simulink model "Project_000481137"  (R2022b)
settings: Solver=VariableStepAuto  StartTime=0.0  StopTime=10.0  RelTol=1e-3
values from neighbouring files (symbols this model uses):
  a1 = 0.3102    [Constants.m]
  A1 = 8.04e-4    (= 0.000804)    [Constants.m]
  a2 = 49.18    [Constants.m]
  A2 = 4.24e-4    (= 0.000424)    [Constants.m]
  a3 = 1.843    [Constants.m]
  Emax = 1.8e9    (= 1800000000)    [Constants.m]
  k = 0.9907    [Constants.m]
  L1 = 1.038e-13    [Constants.m]
  L2 = 8.485e-13    [Constants.m]
  Li = 1.19e-12    [Constants.m]
  omegan = 481.3    [Constants.m]
  Pmax = 2.8e7    (= 28000000)    [Constants.m]
  Pt = 0.3e6    (= 300000)    [Constants.m]
  v01 = 1.07e-4    (= 0.000107)    [Constants.m]
  v02 = 1.07e-4    (= 0.000107)    [Constants.m]
  zeeta = 0.5588    [Constants.m]
libraries: simulink x1
settings Model: Creator=jonil  LastModifiedBy=jonil

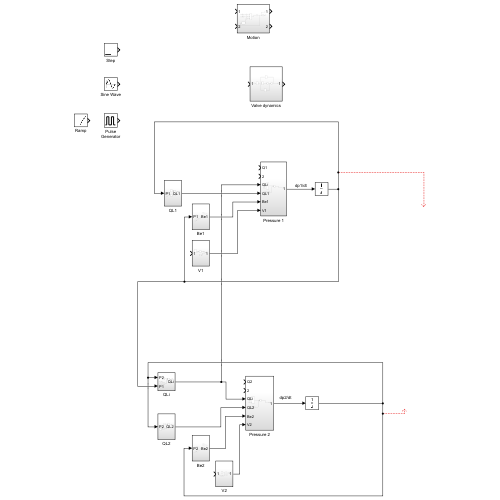
[thumbnail: Simulink's stored preview of the top-level diagram]
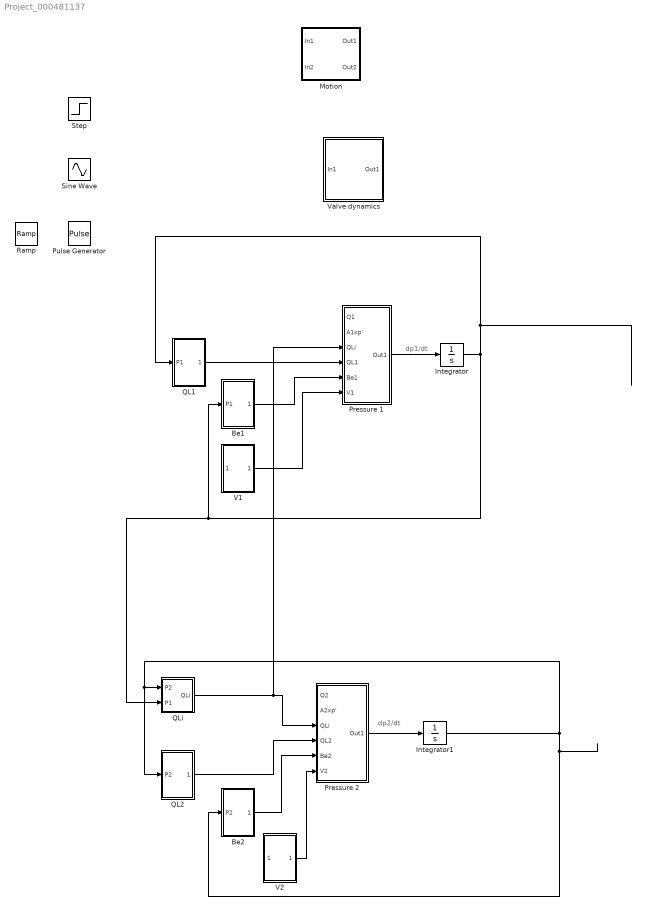
== system Project_000481137 ==
  note: dp2/dt
  note: dp1/dt
  Be1 : Subsystem
  Be2 : Subsystem
  Integrator : Integrator
  Integrator1 : Integrator
  Motion : Subsystem
  Pressure 1 : Subsystem
  Pressure 2 : Subsystem
  Pulse Generator : DiscretePulseGenerator  PulseType=Time based  Period=10  PulseWidth=5
  QL1 : Subsystem
  QL2 : Subsystem
  QLi : Subsystem
  Ramp : simulink/Sources/Ramp  slope=1  start=0  InitialOutput=0
  Sine Wave : Sin  SampleTime=0
  Step : Step  SampleTime=0
  V1 : Subsystem
  V2 : Subsystem
  Valve dynamics : Subsystem
  wires:
  Integrator1/1 -> QL2/1(P2), QLi/1(P2), Be2/1(P2)
  Integrator/1 -> QLi/2(P1), Be1/1(P1), QL1/1(P1)
  QL2/1(QL2) -> Pressure 2/4(QL2)
  Be2/1(Be2) -> Pressure 2/5(Be2)
  V2/1(Out1) -> Pressure 2/6(V2)
  Pressure 2/1(Out1) -> Integrator1/1
  QLi/1(QLi) -> Pressure 1/3(QLi), Pressure 2/3(QLi)
  QL1/1(QL1) -> Pressure 1/4(QL1)
  Be1/1(Be1) -> Pressure 1/5(Be1)
  V1/1(Out1) -> Pressure 1/6(V1)
  Pressure 1/1(Out1) -> Integrator/1

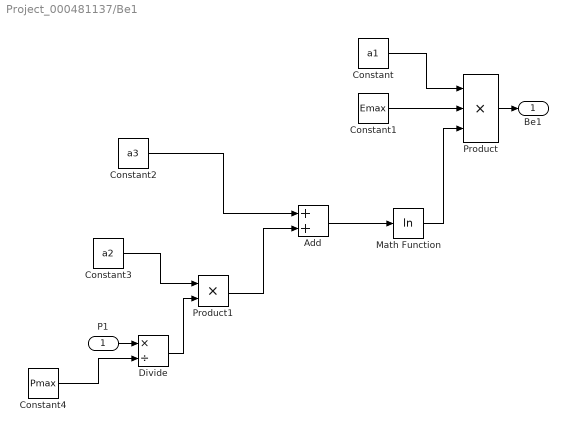
== system Project_000481137/Be1 ==
  P1 : Inport
  Add : Sum
  Constant : Constant  Value=a1
  Constant1 : Constant  Value=Emax
  Constant2 : Constant  Value=a3
  Constant3 : Constant  Value=a2
  Constant4 : Constant  Value=Pmax
  Divide : Product  Inputs=*/
  Math Function : Math  Operator=log
  Product : Product  Inputs=3
  Product1 : Product
  Be1 : Outport
  wires:
  Constant1/1 -> Product/2
  Product/1 -> Be1/1
  Product1/1 -> Add/2
  Constant2/1 -> Add/1
  Math Function/1 -> Product/3
  Constant/1 -> Product/1
  Add/1 -> Math Function/1
  Divide/1 -> Product1/2
  Constant4/1 -> Divide/2
  Constant3/1 -> Product1/1
  P1/1 -> Divide/1

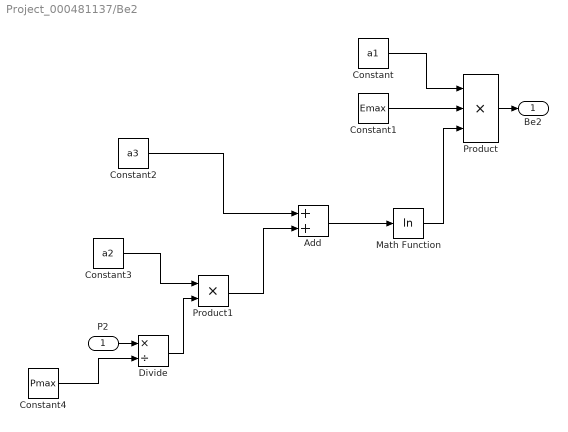
== system Project_000481137/Be2 ==
  P2 : Inport
  Add : Sum
  Constant : Constant  Value=a1
  Constant1 : Constant  Value=Emax
  Constant2 : Constant  Value=a3
  Constant3 : Constant  Value=a2
  Constant4 : Constant  Value=Pmax
  Divide : Product  Inputs=*/
  Math Function : Math  Operator=log
  Product : Product  Inputs=3
  Product1 : Product
  Be2 : Outport
  wires:
  P2/1 -> Divide/1
  Constant3/1 -> Product1/1
  Constant4/1 -> Divide/2
  Divide/1 -> Product1/2
  Add/1 -> Math Function/1
  Constant/1 -> Product/1
  Math Function/1 -> Product/3
  Constant2/1 -> Add/1
  Product1/1 -> Add/2
  Product/1 -> Be2/1
  Constant1/1 -> Product/2

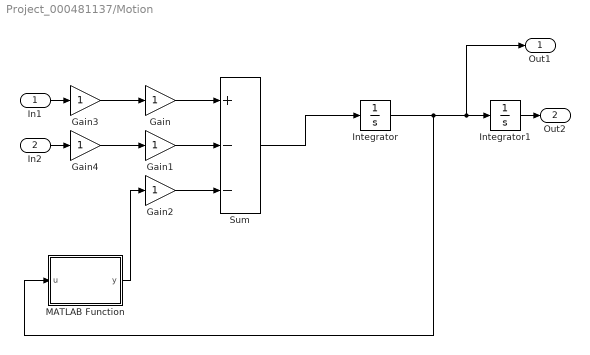
== system Project_000481137/Motion ==
  In1 : Inport
  In2 : Inport  Port=2
  Gain{,1..4} (5 alike) : Gain
  Integrator : Integrator
  Integrator1 : Integrator
  MATLAB Function : MATLAB Function  TreatAsAtomicUnit=on
  Sum : Sum  Inputs=+--
  Out1 : Outport
  Out2 : Outport  Port=2
  wires:
  Gain4/1 -> Gain1/1
  Gain2/1 -> Sum/3
  Gain3/1 -> Gain/1
  Gain1/1 -> Sum/2
  Gain/1 -> Sum/1
  Integrator/1 -> MATLAB Function/1(u), Out1/1, Integrator1/1
  In2/1 -> Gain4/1
  Sum/1 -> Integrator/1
  Integrator1/1 -> Out2/1
  MATLAB Function/1(y) -> Gain2/1
  In1/1 -> Gain3/1

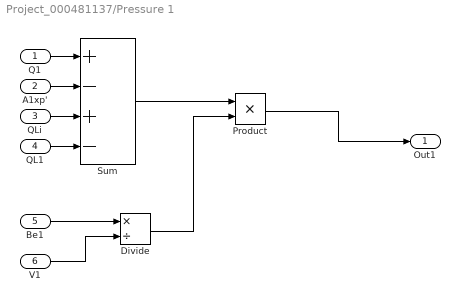
== system Project_000481137/Pressure 1 ==
  Q1 : Inport
  A1xp' : Inport  Port=2
  QLi : Inport  Port=3
  QL1 : Inport  Port=4
  Be1 : Inport  Port=5
  V1 : Inport  Port=6
  Divide : Product  Inputs=*/
  Product : Product
  Sum : Sum  Inputs=+-+-
  Out1 : Outport
  wires:
  Be1/1 -> Divide/1
  QL1/1 -> Sum/4
  Product/1 -> Out1/1
  QLi/1 -> Sum/3
  Q1/1 -> Sum/1
  Sum/1 -> Product/1
  Divide/1 -> Product/2
  A1xp'/1 -> Sum/2
  V1/1 -> Divide/2

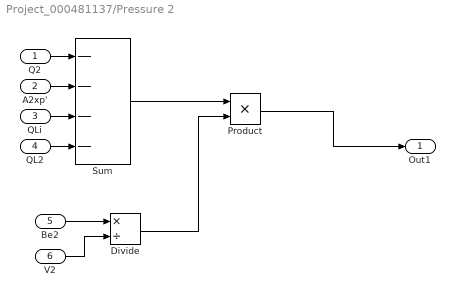
== system Project_000481137/Pressure 2 ==
  Q2 : Inport
  A2xp' : Inport  Port=2
  QLi : Inport  Port=3
  QL2 : Inport  Port=4
  Be2 : Inport  Port=5
  V2 : Inport  Port=6
  Divide : Product  Inputs=*/
  Product : Product
  Sum : Sum  Inputs=----
  Out1 : Outport
  wires:
  A2xp'/1 -> Sum/2
  Divide/1 -> Product/2
  Be2/1 -> Divide/1
  Q2/1 -> Sum/1
  Product/1 -> Out1/1
  Sum/1 -> Product/1
  QLi/1 -> Sum/3
  V2/1 -> Divide/2
  QL2/1 -> Sum/4

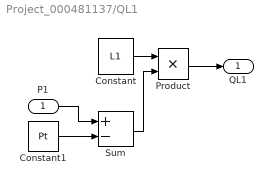
== system Project_000481137/QL1 ==
  P1 : Inport
  Constant : Constant  Value=L1
  Constant1 : Constant  Value=Pt
  Product : Product
  Sum : Sum  Inputs=+-
  QL1 : Outport
  wires:
  Constant/1 -> Product/1
  Sum/1 -> Product/2
  P1/1 -> Sum/1
  Constant1/1 -> Sum/2
  Product/1 -> QL1/1

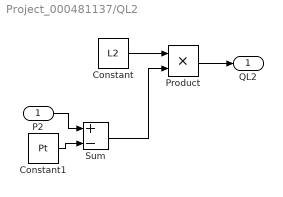
== system Project_000481137/QL2 ==
  P2 : Inport
  Constant : Constant  Value=L2
  Constant1 : Constant  Value=Pt
  Product : Product
  Sum : Sum  Inputs=+-
  QL2 : Outport
  wires:
  Product/1 -> QL2/1
  Constant1/1 -> Sum/2
  P2/1 -> Sum/1
  Sum/1 -> Product/2
  Constant/1 -> Product/1

== system Project_000481137/QLi ==
  P2 : Inport
  P1 : Inport  Port=2
  Constant : Constant  Value=Li
  Product : Product
  Sum : Sum  Inputs=+-
  QLi : Outport
  wires:
  Sum/1 -> Product/2
  Constant/1 -> Product/1
  P1/1 -> Sum/2
  Product/1 -> QLi/1
  P2/1 -> Sum/1

== system Project_000481137/V1 ==
  In1 : Inport
  Pipe Volume1 : Constant  Value=v01
  Piston Area : Constant  Value=A1
  Product : Product
  Sum : Sum
  Out1 : Outport
  wires:
  Sum/1 -> Out1/1
  In1/1 -> Product/2
  Piston Area/1 -> Product/1
  Product/1 -> Sum/1
  Pipe Volume1/1 -> Sum/2

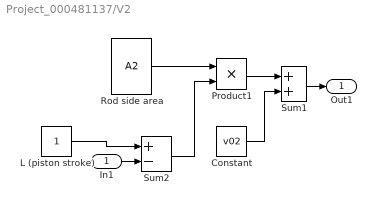
== system Project_000481137/V2 ==
  In1 : Inport
  Constant : Constant  Value=v02
  L (piston stroke) : Constant
  Product1 : Product
  Rod side area : Constant  Value=A2
  Sum1 : Sum
  Sum2 : Sum  Inputs=+-
  Out1 : Outport
  wires:
  Constant/1 -> Sum1/2
  Rod side area/1 -> Product1/1
  Product1/1 -> Sum1/1
  In1/1 -> Sum2/2
  L (piston stroke)/1 -> Sum2/1
  Sum2/1 -> Product1/2
  Sum1/1 -> Out1/1

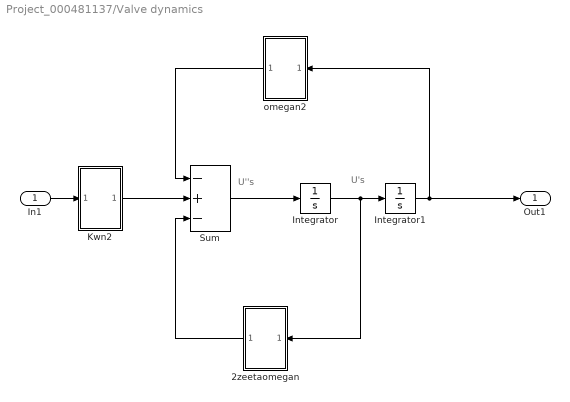
== system Project_000481137/Valve dynamics ==
  note: U''s
  note: U's
  In1 : Inport
  2zeetaomegan : Subsystem
  Integrator : Integrator
  Integrator1 : Integrator
  Kwn2 : Subsystem
  Sum : Sum  Inputs=-+-
  omegan2 : Subsystem
  Out1 : Outport
  wires:
  2zeetaomegan/1(Out1) -> Sum/3
  Sum/1 -> Integrator/1
  Integrator/1 -> 2zeetaomegan/1(In1), Integrator1/1
  Integrator1/1 -> omegan2/1(In1), Out1/1
  In1/1 -> Kwn2/1(In1)
  Kwn2/1(Out1) -> Sum/2
  omegan2/1(Out1) -> Sum/1

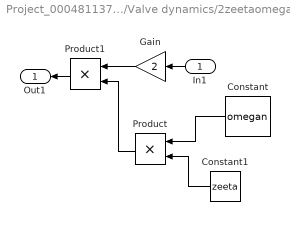
== system Project_000481137/Valve dynamics/2zeetaomegan ==
  In1 : Inport
  Constant : Constant  Value=omegan
  Constant1 : Constant  Value=zeeta
  Gain : Gain  Gain=2
  Product : Product
  Product1 : Product
  Out1 : Outport
  wires:
  Product1/1 -> Out1/1
  Product/1 -> Product1/2
  Gain/1 -> Product1/1
  Constant1/1 -> Product/2
  Constant/1 -> Product/1
  In1/1 -> Gain/1

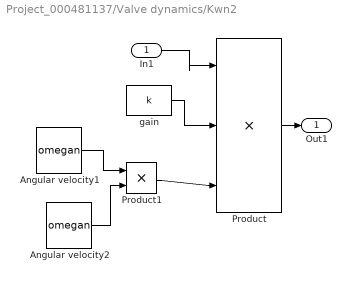
== system Project_000481137/Valve dynamics/Kwn2 ==
  In1 : Inport
  Angular velocity1 : Constant  Value=omegan
  Angular velocity2 : Constant  Value=omegan
  Product : Product  Inputs=3
  Product1 : Product
  gain : Constant  Value=k
  Out1 : Outport
  wires:
  gain/1 -> Product/2
  Angular velocity1/1 -> Product1/1
  Product/1 -> Out1/1
  Product1/1 -> Product/3
  In1/1 -> Product/1
  Angular velocity2/1 -> Product1/2

== system Project_000481137/Valve dynamics/omegan2 ==
  In1 : Inport
  Constant : Constant  Value=omegan
  Constant1 : Constant  Value=omegan
  Product : Product
  Product1 : Product
  Out1 : Outport
  wires:
  Product/1 -> Product1/1
  Constant/1 -> Product/1
  Constant1/1 -> Product/2
  In1/1 -> Product1/2
  Product1/1 -> Out1/1

== matlab function Project_000481137/Motion/MATLAB Function ==
  data: u input; y output
function y = fcn(u)

y = u;
